simulink subsystem "BrakingHydraulics"  (R2023a)
settings: Solver=VariableStepAuto  StartTime=0.0  StopTime=10.0  RelTol=1e-3
undefined symbols (not defined in the file): PlntBrkFrntBias, PlntBrkPrsFctr, PlntBrkRearBias
libraries: autolibutils x1
settings Model: ModifiedByFormat=The MathWorks, Inc.  Creator=The MathWorks, Inc.  LastModifiedBy=The MathWorks, Inc.
settings OptimizationCC: ReuseModelBlockBuffer=off

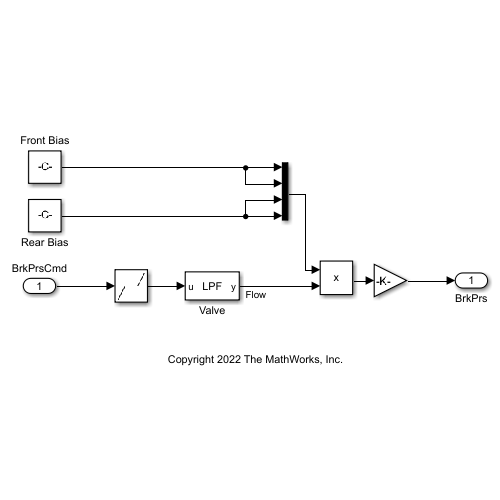
[thumbnail: Simulink's stored preview of the top-level diagram]
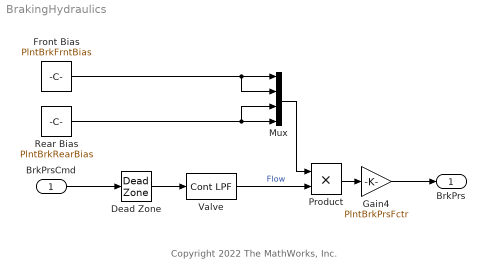
== system BrakingHydraulics ==
  note: Copyright 2022 The MathWorks, Inc.
  BrkPrsCmd : Inport
  Dead Zone : DeadZone  LowerValue=-inf  UpperValue=1e-3  ZeroCross=off
  Front Bias : Constant  Value=PlntBrkFrntBias  SampleTime=-1
  Gain4 : Gain  Gain=PlntBrkPrsFctr
  Mux : Mux
  Product : Product
  Rear Bias : Constant  Value=PlntBrkRearBias  SampleTime=-1
  Valve : autolibutils/Cont LPF  wc=PlntBrkWc  AbsoluteTolerance=auto  aMode=6
  BrkPrs : Outport  VectorParamsAs1DForOutWhenUnconnected=off
  wires:
  Rear Bias/1 -> Mux/3, Mux/4
  Mux/1 -> Product/1
  Dead Zone/1 -> Valve/1
  BrkPrsCmd/1 -> Dead Zone/1
  Product/1 -> Gain4/1
  Front Bias/1 -> Mux/2, Mux/1
  Valve/1 -> Product/2  "Flow"
  Gain4/1 -> BrkPrs/1
